simulink model "BLAC_MotorCtrl_Math"  (R2025b)
settings: Solver=FixedStepDiscrete  StartTime=0.0  StopTime=5  FixedStep=MC_Sim_BaseStep  RelTol=1e-3  EnableMultiTasking=on
values from neighbouring files (symbols this model uses):
  MC_Hardware_Chip_ADCResultBit = 0.0    [MotorControlDataDictionary_Math.sldd]
  MC_Hardware_Chip_ADCVoltageMax = 1.0    [MotorControlDataDictionary_Math.sldd]
  MC_Hardware_Chip_ADCVoltageRefence = 0.0    [MotorControlDataDictionary_Math.sldd]
  MC_Hardware_Chip_CSAGain = 1.0    [MotorControlDataDictionary_Math.sldd]
  MC_Sim_BaseStep = 2.5E-8    [MotorControlDataDictionary_Math.sldd]
  MC_Sim_HFTStep = 6.6675E-5    [MotorControlDataDictionary_Math.sldd]
undefined symbols (not defined in the file or in its folder): MC_MOS_DeadTime, MC_Motor_Phi, MC_Motor_Rotor_Pn, MC_Motor_Stator_Ld, MC_Motor_Stator_Lq, MC_Motor_Stator_Rs, MC_Param_CurrentPI_Ki, MC_Param_CurrentPI_Kp, MC_Param_CurrentPI_UdInteMax, MC_Param_CurrentPI_UdInteMin, MC_Param_CurrentPI_UdMax, MC_Param_CurrentPI_UdMin, MC_Param_CurrentPI_UqInteMax, MC_Param_CurrentPI_UqInteMin, MC_Param_CurrentPI_UqMax, MC_Param_CurrentPI_UqMin, MC_Param_Flux_Gamma, MC_Param_Flux_Lalpha, MC_Param_Flux_Lbeta, MC_Param_Flux_Ralpha, MC_Param_Flux_Rbeta, MC_Param_Luen_BEMFalpha, MC_Param_Luen_BEMFbeta, MC_Param_Luen_BEMFErr, MC_Param_Luen_Currentalpha, MC_Param_Luen_Currentbeta, MC_Param_Luen_CurrentErr, MC_Param_Luen_PLL_Ki, MC_Param_Luen_PLL_Kp, MC_Param_Luen_Voltagealpha, MC_Param_Luen_Voltagebeta, MC_Param_PhasetoReal, MC_Param_SMO_CoffA, MC_Param_SMO_CoffB, MC_Param_SpeedtoTheta, MC_Param_SVPWM_DutyMax, MC_Param_SVPWM_DutyMin, MC_Param_SVPWM_SampleOffset1, MC_Param_SVPWM_SampleOffset2, MC_Param_SVPWM_SampleValid
libraries: simulink x31, nesl_utility x22, ee_lib x21, fl_lib x16, spsSeriesRLCBranchLib x2, spsVoltageMeasurementLib x2
(part 1 of 5)
settings Model: DataDictionary=MotorControlDataDictionary_Math.sldd  SimulationMode=accelerator  Creator=YXuan  LastModifiedBy=YXuan
settings SolverCC: PositivePriorityOrder=on  AutoInsertRateTranBlk=on
settings OptimizationCC: DefaultParameterBehavior=Inlined  EnhancedBackFolding=on  PassReuseOutputArgsAs=Individual arguments  ZeroExternalMemoryAtStartup=off  ZeroInternalMemoryAtStartup=off  OptimizeBlockOrder=speed  DifferentSizesBufferReuse=on  OptimizationCustomize=off  EfficientTunableParamExpr=on
settings DebuggingCC: ParameterTunabilityLossMsg=error
settings SFSimCC: MATLABDynamicMemAlloc=off
settings RTWCC: SystemTargetFile=ert.tlc  TemplateMakefile=ert_default_tmf  GPUComputeCapability=3.5  Description=Embedded Coder
settings CodeAppCC: ForceParamTrailComments=on  IgnoreCustomStorageClasses=off  OperatorAnnotations=on  SimulinkDataObjDesc=on  SFDataObjDesc=on  InsertBlockDesc=on
settings ERTTargetCC: ERTCustomFileTemplate=example_file_process.tlc  DynamicArrayContainerType=coder::array  TargetLangStandard=C99 (ISO)  GenerateSampleERTMain=on

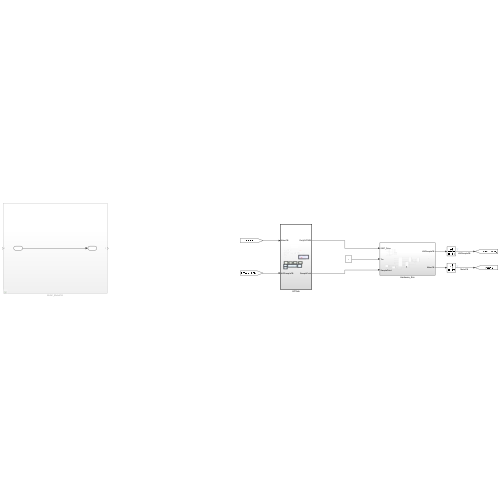
[thumbnail: Simulink's stored preview of the top-level diagram]
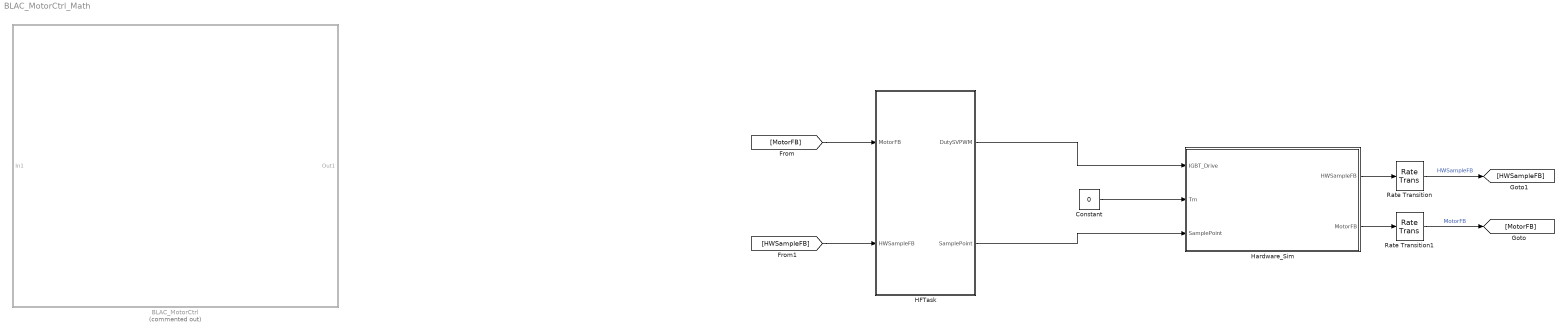
== system BLAC_MotorCtrl_Math ==
  BLAC_MotorCtrl : Subsystem  Commented=on
  Constant : Constant  Value=0
  HFTask : Subsystem  TreatAsAtomicUnit=on  SystemSampleTime=MC_Sim_HFTStep
  Hardware_Sim : Subsystem
  Rate Transition : RateTransition  OutPortSampleTime=MC_Sim_HFTStep
  Rate Transition1 : RateTransition  OutPortSampleTime=MC_Sim_HFTStep
  wires:
  HFTask/1(DutySVPWM) -> Hardware_Sim/1(IGBT_Drive)
  HFTask/2(SamplePoint) -> Hardware_Sim/3(SamplePoint)
  [MotorFB] -> HFTask/1(MotorFB)
  [HWSampleFB] -> HFTask/2(HWSampleFB)
  Constant/1 -> Hardware_Sim/2(Tm)
  Hardware_Sim/2(MotorFB) -> Rate Transition1/1
  Hardware_Sim/1(HWSampleFB) -> Rate Transition/1
  Rate Transition/1 -> [HWSampleFB]  "HWSampleFB"
  Rate Transition1/1 -> [MotorFB]  "MotorFB"

== system BLAC_MotorCtrl_Math/BLAC_MotorCtrl ==
  In1 : Inport
  Out1 : Outport
  wires:
  In1/1 -> Out1/1

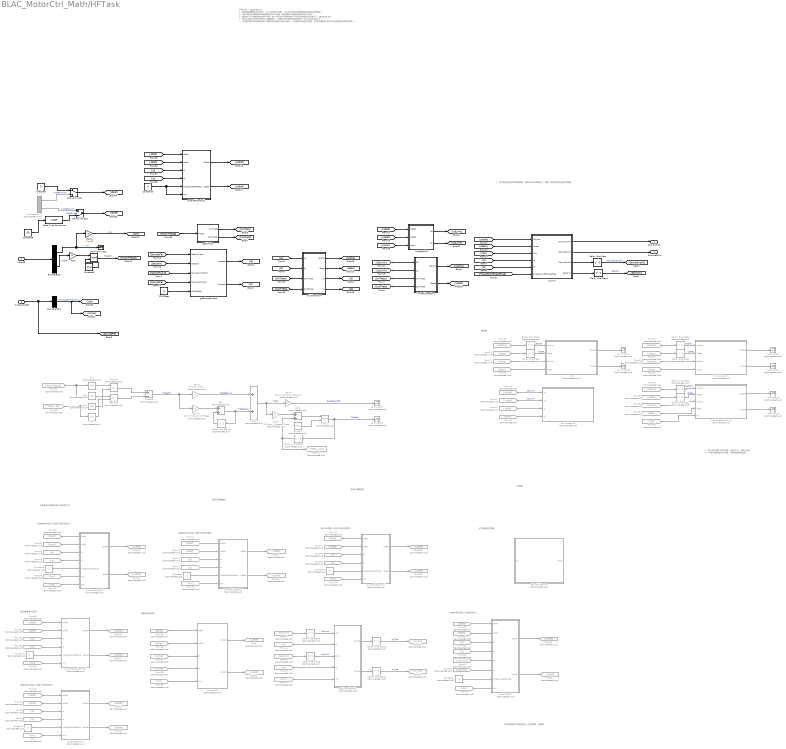
== system BLAC_MotorCtrl_Math/HFTask ==
  note: 待更新电压控制的积分抗饱和方式
  note: 传统电流PI控制（前馈+电流抗饱和）
  note: 1、PLL存在问题(带宽问题，10hz可以，50hz溢出)
      | 2、方程反馈参数存在问题，导致观测角度超前
  note: 观测器
  note: 无差拍电流控制
  note: 开发日志：
      | 2025.03.24:
      | 1、磁链观测器增益应该适中（过小会导致不收敛，过大则会导致观测角度相位超前实际角度）
      | 2、无差拍电流控制是否采用预测电流进行控制？是否要进行旋转反电势的电压补偿？
      | 3、静态电压补偿模型增益如何设置？输入电压是采用理想电压还是采样的电机实际电压？
      | 2025.03.25:
      | 1、测试发现电压和电流呈现2个周期延时，无差拍应考虑做电流预测两个节拍
      | 2025.03.27：
      | 1、无差拍控制应采用延时两个周期的电流和电压进行延时一个周期的电流进行预测，然后用预测电流作为电流控制的反馈电流输入。
      | 2025.12.13:
      | 1、增加真实相电压计算（待添加）
      | 2、考虑MPTA、弱磁、以及MPTV模块的防止位置
      | 2026.01.01：
      | 1、增加卡尔曼滤波模块（未构建）
      | 2、增加PIR控制器（未整定参数）
      | 2026.01.28：
      | 1、发现ADRC的电流观测值初期收敛速度较慢，并且存在稳定的误差。
  note: 复矢量电流PI控制
  note: 传统电流PI控制（前馈+电压抗饱和）
  note: ADRC电流控制（性能待优化）
  note: 传统电流PID控制（前馈+电流抗饱和）
  note: 待进行参数整定
  note: 电流PIR控制（前馈+电流抗饱和）
  note: 待进行参数整定
  note: 卡尔曼滤波观测器
  note: 待构建
  note: 1、优化的单电阻采样移相策略、增加单边采样策略
      | 2、增加三电阻和两电阻采样策略
  note: 电流观测值与实际值存在一定的误差，待解决
  MotorFB : Inport
  HWSampleFB : Inport  Port=2
  Add : Sum  Commented=on
  Add1 : Sum  Commented=on
  Add2 : Sum  Commented=on
  Bus Selector : BusSelector  OutputSignals=w,theta
  Bus Selector1 : BusSelector  OutputSignals=Vbus_Sample_DC
  Bus Selector3 : BusSelector  Commented=on  OutputSignals=IdRefLimit,IqRefLimit
  CSAOffset : Constant  Value=0  OutDataTypeStr=single
  Constant : Constant  Commented=on  Value=2*pi  OutDataTypeStr=single
  Constant{1..5,7} (6 alike) : Constant  Commented=on  Value=0  OutDataTypeStr=boolean
  Constant6 : Constant  Value=2*pi  OutDataTypeStr=single
  Constant8 : Constant  Value=50
  Constant9 : Constant  Value=0  OutDataTypeStr=boolean
  Data Type Conversion : DataTypeConversion  OutDataTypeStr=single  RndMeth=Simplest  SaturateOnIntegerOverflow=off
  Delay One Step : Delay
  Delay One Step1 : Delay
  Delay One Step{8..11} (4 alike) : Delay  Commented=on  DelayLength=1
  Delay One Step12 : Delay  Commented=on  DelayLength=0
  Delay One Step13 : Delay  Commented=on  DelayLength=0
  Delay One Step{2..7} (6 alike) : Delay  Commented=on
  From{,39,46,59,70,75} (6 alike) : From  Commented=on  GotoTag=Wm
  From{10,35,42,50,60,66,71,76} (8 alike) : From  Commented=on  GotoTag=IdRef
  From{11,36,43,51,61,67,72,77} (8 alike) : From  Commented=on  GotoTag=IqRef
  From{2,44,52,62,68,73,78} (7 alike) : From  Commented=on  GotoTag=Id
  From25 : From  Commented=on  GotoTag=Ualpha
  From26 : From  Commented=on  GotoTag=Ubeta
  From27 : From  Commented=on  GotoTag=Ialpha
  From28 : From  Commented=on  GotoTag=Ibeta
  From{3,45,53,63,69,74,79} (7 alike) : From  Commented=on  GotoTag=Iq
  From31 : From  Commented=on  GotoTag=Ualpha
  From32 : From  Commented=on  GotoTag=Ubeta
  From33 : From  Commented=on  GotoTag=Ialpha
  From34 : From  Commented=on  GotoTag=Ibeta
  From37 : From  Commented=on  GotoTag=Id_Pre
  From38 : From  Commented=on  GotoTag=Iq_Pre
  From40 : From  Commented=on  GotoTag=UdRef
  From41 : From  Commented=on  GotoTag=UqRef
  From47 : From  Commented=on  GotoTag=UdLimit
  From48 : From  Commented=on  GotoTag=UqLimit
  From49 : From  Commented=on  GotoTag=We
  From54 : From  Commented=on  GotoTag=Ualpha
  From55 : From  Commented=on  GotoTag=Ubeta
  From56 : From  Commented=on  GotoTag=Ialpha
  From57 : From  Commented=on  GotoTag=Ibeta
  From58 : From  Commented=on  GotoTag=We
  From64 : From  Commented=on  GotoTag=Vdq
  From65 : From  Commented=on  GotoTag=We
  From80 : From  Commented=on  GotoTag=UdLimit
  From81 : From  Commented=on  GotoTag=UqLimit
  From82 : From  Commented=on  GotoTag=Theta_Last
  From83 : From  Commented=on  GotoTag=MotorThetaE
  Gain : Gain  Gain=4  OutDataTypeStr=single
  Gain2 : Gain  Gain=4*pi/30
  Gain3 : Gain  Commented=on  Gain=2*sqrt(2)/2*100
  Gain4 : Gain  Commented=on  Gain=100^2*MC_Sim_HFTStep
  Gain5 : Gain  Commented=on  Gain=MC_Param_SpeedtoTheta  OutDataTypeStr=single  RndMeth=Simplest
  Gain6 : Gain  Commented=on  Gain=30/(pi*MC_Motor_Rotor_Pn)  OutDataTypeStr=single  RndMeth=Simplest
  Goto{,14,30,32,35,37,39} (7 alike) : Goto  Commented=on  GotoTag=UdRef
  Goto{10,26..27,31,34,36,38} (7 alike) : Goto  Commented=on  GotoTag=UqRef
  Goto28 : Goto  Commented=on  GotoTag=Id_Pre
  Goto29 : Goto  Commented=on  GotoTag=Iq_Pre
  Goto40 : Goto  Commented=on  GotoTag=Theta_Last
  Idref_Test : Constant  Value=0  OutDataTypeStr=single
  LuenbergerObservor : Subsystem  Commented=on
  Manual Switch : ManualSwitch
  Manual Switch1 : ManualSwitch  CurrentSetting=0
  Mod : Math  Operator=mod
  Mod1 : Math  Commented=on  Operator=mod
  Product : Product  Commented=on
  Product1 : Product  Commented=on
  Sin : Trigonometry  Commented=on  OutputSignalType=real
  Sin1 : Trigonometry  Commented=on  Operator=cos  OutputSignalType=real
  Sin2 : Trigonometry  Commented=on  OutputSignalType=real
  Sin3 : Trigonometry  Commented=on  Operator=cos  OutputSignalType=real
  Subtract : Sum  Commented=on  Inputs=+-
  Terminator : Terminator
  Terminator{1..8} (8 alike) : Terminator  Commented=on
  axisTransform : Subsystem
  currentADRC : Subsystem  Commented=on
  currentComplexPICtrl : Subsystem  Commented=on
  currentDBC : Subsystem  Commented=on
  currentPIControl : Subsystem  Commented=on
  currentPIControl1 : Subsystem  Commented=on
  currentPIControl2 : Subsystem
  currentPIDControl : Subsystem  Commented=on
  currentPIRControl : Subsystem  Commented=on
  fluxobservor : Subsystem  Commented=on
  getCurrentPredict : Subsystem  Commented=on
  getPhaseCurrent : Subsystem
  getSinCos : Subsystem
  invParkTransform : Subsystem
  karmalObservor : Subsystem  Commented=on
  scvmobservor : Subsystem  Commented=on
  smo : Subsystem  Commented=on
  svpwm : Subsystem  TreatAsAtomicUnit=on
  voltageLimit : Subsystem
  DutySVPWM : Outport
  SamplePoint : Outport  Port=2
  wires:
  Delay One Step2/1 -> smo/1(Valpha)  "Ualpha"
  From25/1 -> Delay One Step2/1
  Delay One Step3/1 -> smo/2(Vbeta)  "Ubeta"
  From26/1 -> Delay One Step3/1
  From27/1 -> smo/3(Ialpha)
  From28/1 -> smo/4(Ibeta)
  smo/1(Speed) -> Terminator2/1
  smo/2(Theta) -> Terminator3/1
  [PhaseShortEnableFlag] -> svpwm/6(PhaseShortEnableFlag)
  [Umax] -> voltageLimit/3(Umax)
  svpwm/4(SectorN) -> Delay One Step1/1
  axisTransform/2(Ibeta) -> [Ibeta]
  svpwm/3(SampleValid) -> Delay One Step/1
  svpwm/1(DutySVPWM) -> DutySVPWM/1
  [SampleFB] -> getPhaseCurrent/4(SampleCurrent)
  [SectorN] -> getPhaseCurrent/2(SectorN)
  [UdRef] -> voltageLimit/1(UdRef)
  [UdLimit] -> invParkTransform/1(Ud)
  currentPIControl/1(UdRef) -> Goto14/1
  [Ubeta] -> svpwm/2(Vbeta)
  axisTransform/1(Ialpha) -> [Ialpha]
  [UqRef] -> voltageLimit/2(UqRef)
  [Ualpha] -> svpwm/1(Valpha)
  [Ia] -> axisTransform/1(Ia)
  svpwm/2(SamplePoint) -> SamplePoint/1
  currentPIControl/2(UqRef) -> Goto10/1
  [Vdc] -> svpwm/3(Vdc)
  voltageLimit/1(Ud) -> [UdLimit]
  [MotorThetaE] -> getSinCos/1(Theta)
  From2/1 -> currentPIControl/3(Id)
  getSinCos/1(SinTheta) -> [SinTheta]
  [SampleValid] -> getPhaseCurrent/3(SampleValid[2])
  axisTransform/3(Id) -> [Id]
  getPhaseCurrent/2(Ibselect) -> [Ib]
  From/1 -> currentPIControl/6(Wm)
  axisTransform/4(Iq) -> [Iq]
  From3/1 -> currentPIControl/4(Iq)
  Constant2/1 -> currentPIControl/5(IntregralResetFlag)
  [Ib] -> axisTransform/2(Ib)
  [UqLimit] -> invParkTransform/2(Uq)
  [SinTheta] -> invParkTransform/3(SinTheta)
  Delay One Step1/1 -> [SectorN]  "SectorN"
  [CosTheta] -> invParkTransform/4(CosTheta)
  invParkTransform/1(Ualpha) -> [Ualpha]
  Delay One Step/1 -> [SampleValid]  "SampleValid[2]"
  getSinCos/2(CosTheta) -> [CosTheta]
  voltageLimit/2(Uq) -> [UqLimit]
  [SinTheta] -> axisTransform/3(SinTheta)
  getPhaseCurrent/1(Iaselect) -> [Ia]
  CSAOffset/1 -> getPhaseCurrent/5(CSAOffset)
  [CosTheta] -> axisTransform/4(CosTheta)
  invParkTransform/2(Ubeta) -> [Ubeta]
  [Ib] -> svpwm/5(Ib)
  [Ia] -> svpwm/4(Ia)
  Bus Selector/2 -> Gain/1  "<theta>"
  Bus Selector/1 -> Terminator/1, Gain2/1  "<w>"
  Mod/1 -> [MotorThetaE]  "ThetaE"
  Gain/1 -> Mod/1
  HWSampleFB/1 -> [SampleFB], Bus Selector1/1
  Constant6/1 -> Mod/2
  MotorFB/1 -> Bus Selector/1
  From10/1 -> currentPIControl/1(IdRef)
  From11/1 -> currentPIControl/2(IqRef)
  From34/1 -> fluxobservor/4(Ibeta)
  From33/1 -> fluxobservor/3(Ialpha)
  From32/1 -> Delay One Step5/1
  From31/1 -> Delay One Step4/1
  Delay One Step4/1 -> fluxobservor/1(Valpha)  "Ualpha"
  Delay One Step5/1 -> fluxobservor/2(Vbeta)  "Ubeta"
  fluxobservor/1(Speed) -> Terminator1/1
  fluxobservor/2(Theta) -> Terminator4/1
  currentDBC/2(UqRef) -> Goto26/1
  From36/1 -> currentDBC/2(IqRef)
  From35/1 -> currentDBC/1(IdRef)
  From37/1 -> currentDBC/3(Id)
  From38/1 -> currentDBC/4(Iq)
  From39/1 -> currentDBC/5(Wm)
  From41/1 -> scvmobservor/2(Vq)  "UqLimit"
  From40/1 -> scvmobservor/1(Vd)  "UdLimit"
  From42/1 -> scvmobservor/3(Id)
  From43/1 -> scvmobservor/4(Iq)
  Gain2/1 -> [We]  "We"
  From44/1 -> getCurrentPredict/2(Id)
  From45/1 -> getCurrentPredict/4(Iq)
  From46/1 -> getCurrentPredict/5(Wm)
  From47/1 -> Delay One Step8/1
  From48/1 -> Delay One Step9/1
  getCurrentPredict/1(Id_Pre) -> Delay One Step12/1
  getCurrentPredict/2(Iq_Pre) -> Delay One Step13/1
  currentDBC/1(UdRef) -> Goto/1
  Delay One Step8/1 -> getCurrentPredict/1(Ud1)  "UdLimit"
  Delay One Step9/1 -> getCurrentPredict/3(Uq1)  "UqLimit"
  Delay One Step12/1 -> Goto28/1  "Id_Pre"
  Delay One Step13/1 -> Goto29/1  "Iq_Pre"
  From51/1 -> currentComplexPICtrl/2(IqRef)
  From50/1 -> currentComplexPICtrl/1(IdRef)
  Constant1/1 -> currentComplexPICtrl/5(IntregralResetFlag)
  From53/1 -> currentComplexPICtrl/4(Iq)
  From49/1 -> currentComplexPICtrl/6(Wm)
  From52/1 -> currentComplexPICtrl/3(Id)
  currentComplexPICtrl/2(UqRef) -> Goto27/1
  currentComplexPICtrl/1(UdRef) -> Goto30/1
  LuenbergerObservor/1(Speed) -> Terminator5/1
  LuenbergerObservor/2(Theta) -> Terminator6/1
  From57/1 -> LuenbergerObservor/4(Ibeta)
  From56/1 -> LuenbergerObservor/3(Ialpha)
  From55/1 -> Delay One Step7/1
  From54/1 -> Delay One Step6/1
  Delay One Step7/1 -> LuenbergerObservor/2(Vbeta)  "Ubeta"
  Delay One Step6/1 -> LuenbergerObservor/1(Valpha)  "Ualpha"
  From58/1 -> LuenbergerObservor/5(We)
  From61/1 -> currentPIControl1/2(IqRef)
  From60/1 -> currentPIControl1/1(IdRef)
  Constant3/1 -> currentPIControl1/5(IntregralResetFlag)
  From63/1 -> currentPIControl1/4(Iq)
  From59/1 -> currentPIControl1/6(Wm)
  From62/1 -> currentPIControl1/3(Id)
  currentPIControl1/2(UqRef) -> Goto31/1
  currentPIControl1/1(UdRef) -> Goto32/1
  From64/1 -> currentPIControl1/7(Vdq)
  currentADRC/1(UdRef) -> Goto35/1
  currentADRC/2(UqRef) -> Goto34/1
  From68/1 -> currentADRC/3(Id)
  From65/1 -> currentADRC/8(Wm)
  From69/1 -> currentADRC/4(Iq)
  Constant4/1 -> currentADRC/7(IntregralResetFlag)
  From66/1 -> currentADRC/1(IdRef)
  From67/1 -> currentADRC/2(IqRef)
  Constant5/1 -> currentPIDControl/5(IntregralResetFlag)
  From71/1 -> currentPIDControl/1(IdRef)
  currentPIDControl/1(UdRef) -> Goto37/1
  From73/1 -> currentPIDControl/3(Id)
  From72/1 -> currentPIDControl/2(IqRef)
  currentPIDControl/2(UqRef) -> Goto36/1
  From70/1 -> currentPIDControl/6(Wm)
  From74/1 -> currentPIDControl/4(Iq)
  Bus Selector3/1 -> Manual Switch/2  "<IdRefLimit>"
  Bus Selector3/2 -> Manual Switch1/1  "<IqRefLimit>"
  Manual Switch/1 -> [IdRef]
  Idref_Test/1 -> Manual Switch/1
  Manual Switch1/1 -> [IqRef]
  Data Type Conversion/1 -> Manual Switch1/2  "IqRef_Test"
  From79/1 -> currentPIRControl/4(Iq)
  From75/1 -> currentPIRControl/6(Wm)
  currentPIRControl/2(UqRef) -> Goto38/1
  From77/1 -> currentPIRControl/2(IqRef)
  From78/1 -> currentPIRControl/3(Id)
  currentPIRControl/1(UdRef) -> Goto39/1
  From76/1 -> currentPIRControl/1(IdRef)
  Constant7/1 -> currentPIRControl/5(IntregralResetFlag)
  From80/1 -> currentADRC/5(Ud)
  From81/1 -> currentADRC/6(Uq)
  Gain5/1 -> Add2/1
  Delay One Step10/1 -> Add/2
  Constant/1 -> Mod1/2
  Mod1/1 -> Terminator8/1, Delay One Step11/1  "ThetaPI"
  Delay One Step11/1 -> Goto40/1, Add2/2
  Gain3/1 -> Add1/1  "ThetaErr_Kp"
  Add1/1 -> Gain6/1, Gain5/1  "WePI"
  Add2/1 -> Mod1/1
  Gain6/1 -> Terminator7/1  "SpeedPI_RPM"
  Subtract/1 -> Gain3/1, Gain4/1  "ThetaErr"
  Add/1 -> Add1/2, Delay One Step10/1  "ThetaErr_Ki"
  Gain4/1 -> Add/1
  From83/1 -> Sin1/1, Sin/1
  From82/1 -> Sin2/1, Sin3/1
  Sin/1 -> Product/1
  Sin3/1 -> Product/2
  Product/1 -> Subtract/1
  Sin1/1 -> Product1/1
  Sin2/1 -> Product1/2
  Product1/1 -> Subtract/2
  Constant8/1 -> Data Type Conversion/1
  [SampleFB] -> getPhaseCurrent/1(RealCurrent)
  Bus Selector1/1 -> [Umax], [Vdc]  "<Vbus_Sample_DC>"
  [IqRef] -> currentPIControl2/2(IqRef)
  [IdRef] -> currentPIControl2/1(IdRef)
  [Iq] -> currentPIControl2/4(Iq)
  [Id] -> currentPIControl2/3(Id)
  currentPIControl2/2(UqRef) -> [UqRef]
  currentPIControl2/1(UdRef) -> [UdRef]
  Constant9/1 -> currentPIControl2/6(Wm), currentPIControl2/5(IntregralResetFlag)

== system BLAC_MotorCtrl_Math/Hardware_Sim ==
  IGBT_Drive : Inport
  Tm : Inport  Port=2
  SamplePoint : Inport  Port=3
  ActoDC_Sim : Subsystem
      settings: PortSchema="{\"entries\":[{\"content\":{\"sides\":[{\"content\":{},\"type\":\"ConnectorPlacement.EquallySpacedRectSide\",\"uuid\":\"dfb3aeea-336c-446c-ad65-e2bc7f8ca636\"},{\"content\":{\"connectorIds\":[\"RConn1\",\"RConn2\",\"RConn3\",\"RConn4\"],\"side\":\"RIGHT\"},\"type\":\"ConnectorPlacement.EquallySpacedRectSide\",\"uuid\":\"0d159b54-293a-4c78-aa60-b1815773a2e6\"},{\"content\":{\"side\":\"TOP\"},\"type\":\"ConnectorPlacement.EquallySpacedRectSide\",\"uuid\":\"3a8a1089-02f9-49de-abe1-3c0c9b1c30b4\"},{\"content\":{\"connectorIds\":[\"RConn5\"],\"side\":\"BOTTOM\"},\"type\":\"ConnectorPlacement.EquallySpacedRectSide\",\"uuid\":\"d5f8019e-9277-4fe4-88e1-78a5ead24f5f\"}]},\"type\":\"ConnectorPlacement.EquallySpacedConnector\",\"uuid\":\"60ec8383-903f-4624-bd14-64a171abc59f\"}],\"packageUris\":[\"http://schema.mathworks.com/mf0/Connector/R2020b\"],\"version\":\"1.0\"}"
  CurrentSample_Sim : Subsystem
      settings: PortSchema="{\"entries\":[{\"content\":{\"sides\":[{\"content\":{\"connectorIds\":[\"LConn1\",\"LConn2\",\"LConn3\"]},\"type\":\"ConnectorPlacement.EquallySpacedRectSide\",\"uuid\":\"6ff7a8d3-c405-46c2-bb14-4046cb7aeae7\"},{\"content\":{\"connectorIds\":[\"Out1\"],\"side\":\"RIGHT\"},\"type\":\"ConnectorPlacement.EquallySpacedRectSide\",\"uuid\":\"30142a9b-9a7e-41fc-b1d2-e3039139c6ca\"},{\"content\":{\"connectorIds\":[\"In1\"],\"side\":\"TOP\"},\"type\":\"ConnectorPlacement.EquallySpacedRectSide\",\"uuid\":\"3160108e-a18c-4d1a-9078-164fb8c05fb9\"},{\"content\":{\"connectorIds\":[\"RConn1\"],\"side\":\"BOTTOM\"},\"type\":\"ConnectorPlacement.EquallySpacedRectSide\",\"uuid\":\"3a8083c0-8ece-4c47-8031-bf566ef0bce5\"}]},\"type\":\"ConnectorPlacement.EquallySpacedConnector\",\"uuid\":\"b4e632a6-7f3d-4ba3-a4f0-ad8004e8ab56\"}],\"packageUris\":[\"http://schema.mathworks.com/mf0/Connector/R2020b\"],\"version\":\"1.0\"}"
  DrivePWM_Sim : Subsystem
  IGBT_Inverter_Sim : Subsystem
  Motor_Machine_Sim : Subsystem
  PMSM : ee_lib/Electromechanical/Permanent Magnet/PMSM  port_option=ee.enum.threePhasePort.expanded  winding_type=ee.enum.electromech.statorconfiguration.wye  machine_param=ee.enum.pmsm.parameterization.constant  nPolePairs=6  pmflux_param=ee.enum.pmflux.fluxlinkage  pm_flux_linkage=0.03 Wb  torque_constant=0.18 N*m/A  back_emf_constant=0.18 V*s/rad  stator_param=ee.enum.statorparam.LdLqL0  Ld=0.00019 H  Lq=0.00025 H  idVec=[-200, 0, 200] A  iqVec=[-200, 0, 200] A  LdMatrix=0.0002 * ones(3, 3) H  LqMatrix=0.0002 * ones(3, 3) H  PmMatrix=0.1 * ones(3, 3) Wb  ktMatrix=0.18 * ones(3, 3) N*m/A  keMatrix=0.18 * ones(3, 3) V*s/rad  L0=0.00016 H  Ls=0.0002 H  Lm=-0.00002 H  Ms=0.00002 H  Rs=0.013 Ohm  zero_sequence=ee.enum.park.zerosequence.include  axes_param=ee.enum.rotorangle.daxis  loss_param=ee.enum.ironloss.none  losses_oc=[0, 0, 0] W  losses_sc=[0, 0, 0] W  f_losses=60 Hz  Isc_losses=95 A  J=0.01 kg*m^2  lam=0 N*m*s/rad  i_d_specify=off  i_d_priority=None  i_d=0 A  i_d_nominal_specify=off  i_d_nominal_value=1  i_d_nominal_unit=A  i_q_specify=off  i_q_priority=None  i_q=0 A  i_q_nominal_specify=off  i_q_nominal_value=1  i_q_nominal_unit=A  torque_specify=off  torque_priority=None  torque=0 N*m  torque_nominal_specify=off  torque_nominal_value=1  torque_nominal_unit=N*m  angular_velocity_specify=off  angular_velocity_priority=High  angular_velocity=0 rpm  angular_velocity_nominal_specify=off  angular_velocity_nominal_value=1  angular_velocity_nominal_unit=rpm  angular_position_specify=off  angular_position_priority=High  angular_position=0 deg  angular_position_nominal_specify=off  angular_position_nominal_value=1  angular_position_nominal_unit=deg  alpha=3.93e-3 1/K  alpha_flux=-0.001 1/K  Tmeas=298.15 K  stator_thermal_mass=100 J/K  rotor_thermal_mass=200 J/K  Rm_percent_rotor=90  Rd_percent_rotor=30  temperatureA_specify=off  temperatureA_priority=High  temperatureA=25 degC  temperatureA_nominal_specify=off  temperatureA_nominal_value=1  temperatureA_nominal_unit=degC  temperatureB_specify=off  temperatureB_priority=High  temperatureB=25 degC  temperatureB_nominal_specify=off  temperatureB_nominal_value=1  temperatureB_nominal_unit=degC  temperatureC_specify=off  temperatureC_priority=High  temperatureC=25 degC  temperatureC_nominal_specify=off  temperatureC_nominal_value=1  temperatureC_nominal_unit=degC  temperatureR_specify=off  temperatureR_priority=High  temperatureR=25 degC  temperatureR_nominal_specify=off  temperatureR_nominal_value=1  temperatureR_nominal_unit=degC
      settings: InternalSimscapePortConfiguration="{\"Bottom\":[],\"Left\":[{\"id\":\"a\",\"label\":\"a\",\"type\":\"foundation.electrical.electrical\"},{\"id\":\"b\",\"label\":\"b\",\"type\":\"foundation.electrical.electrical\"},{\"id\":\"c\",\"label\":\"c\",\"type\":\"foundation.electrical.electrical\"},{\"id\":\"n\",\"label\":\"n\",\"type\":\"foundation.electrical.electrical\"}],\"Right\":[{\"id\":\"R\",\"label\":\"R\",\"type\":\"foundation.mechanical.rotational.rotational\"},{\"id\":\"C\",\"label\":\"C\",\"type\":\"foundation.mechanical.rotational.rotational\"}],\"Top\":[]}"
  Repeating Sequence : simulink/Sources/Repeating Sequence  rep_seq_t=[0 MC_Sim_HFTStep/2 MC_Sim_HFTStep]  rep_seq_y=[0 1 0]
  SampleTrigger_Sim : Subsystem
  Solver Configuration : nesl_utility/Solver Configuration  PhysicalDomain=network_engine_domain  SubClassName=solver  LeftPortType=input  RightPortType=generic  Tones=[]  Harmonics=[]  SimulateNoise=off  Profile=off  UseLocalSampling=off  EnableSwitchedLinearOptims=on  FrequencyDomain=off  UseCCode=off  RelTol=0.001  AbsTol=0.001  MinStep=1e-09  ToWorkspace=off  RevertToSquareIcSolve=off  NumHomotopyIterations=100  PhasorMode=off  PhasorModeNumHarmonics=1  ConsistencySolver=NEWTON_XTOL_AFTER_FTOL  IndexReductionMethod=DerivativeReplacement  DoDC=off  ResidualTolerance=1e-09  ConsistencyTolSource=GLOBAL  ConsistencyAbsTol=0.001  ConsistencyRelTol=0.001  ConsistencyTolFactor=0.001  UseLocalSolver=off  LocalSolverChoice=NE_BACKWARD_EULER_ADVANCER  ResolveIndetEquations=on  FunctionEvalNumThread=1  LocalSolverSampleTime=0.001  DoFixedCost=off  MaxNonlinIter=3  MaxModeIter=2  ComputeImpulses=off  ImpulseIterations=2  LinearAlgebra=auto  LinearAlgebraNumThread=0  EquationFormulation=NE_TIME_EF  DelaysMemoryBudget=1024  AutomaticFiltering=on  FilteringTimeConstant=0.001  PartitionStorageMethod=AS_NEEDED  PartitionMemoryBudget=1024  PartitionMethod=ROBUST  MultibodyUseLocalSolver=off  MultibodyLocalSolverChoice=ODE1  MultibodyLocalSolverSampleTime=0.001
  Subsystem : Subsystem
      settings: PortSchema="{\"entries\":[{\"content\":{\"sides\":[{\"content\":{\"connectorIds\":[\"LConn1\",\"LConn2\",\"LConn3\"]},\"type\":\"ConnectorPlacement.EquallySpacedRectSide\",\"uuid\":\"af0e302a-6fe8-4ee5-ad7b-36fa2462e52a\"},{\"content\":{\"connectorIds\":[\"Out1\",\"Out2\",\"Out3\",\"RConn1\",\"RConn2\",\"RConn3\",\"RConn4\"],\"side\":\"RIGHT\"},\"type\":\"ConnectorPlacement.EquallySpacedRectSide\",\"uuid\":\"81cc88e0-41b7-4998-ab4b-7cd10d736f31\"},{\"content\":{\"side\":\"TOP\"},\"type\":\"ConnectorPlacement.EquallySpacedRectSide\",\"uuid\":\"a12e26d5-ba08-4fd7-9848-733d0ad7d51d\"},{\"content\":{\"connectorIds\":[\"RConn5\"],\"side\":\"BOTTOM\"},\"type\":\"ConnectorPlacement.EquallySpacedRectSide\",\"uuid\":\"d3c07252-42de-4432-99bf-cb622f01e596\"}]},\"type\":\"ConnectorPlacement.EquallySpacedConnector\",\"uuid\":\"b6ff19e2-c175-4441-b83d-f6984fbd2671\"}],\"packageUris\":[\"http://schema.mathworks.com/mf0/Connector/R2020b\"],\"version\":\"1.0\"}"
  VbusSample_Sim : Subsystem
      settings: PortSchema="{\"entries\":[{\"content\":{\"sides\":[{\"content\":{\"connectorIds\":[\"LConn1\",\"LConn2\",\"LConn3\",\"LConn4\"]},\"type\":\"ConnectorPlacement.EquallySpacedRectSide\",\"uuid\":\"516f667a-d28d-4d7e-bf09-1844ec397ca8\"},{\"content\":{\"connectorIds\":[\"Out1\",\"Out2\"],\"side\":\"RIGHT\"},\"type\":\"ConnectorPlacement.EquallySpacedRectSide\",\"uuid\":\"8e4c85e3-3d11-4eb4-88a0-2693c28d829e\"},{\"content\":{\"connectorIds\":[\"In1\"],\"side\":\"TOP\"},\"type\":\"ConnectorPlacement.EquallySpacedRectSide\",\"uuid\":\"147b6efa-5ce1-4794-b48d-7dda172e67f0\"}]},\"type\":\"ConnectorPlacement.EquallySpacedConnector\",\"uuid\":\"ecacdeaf-2c45-44a5-a2ad-63e6b49d0bd0\"}],\"packageUris\":[\"http://schema.mathworks.com/mf0/Connector/R2020b\"],\"version\":\"1.0\"}"
  HWSampleFB : Outport
  MotorFB : Outport  Port=2
  wires:
  CurrentSample_Sim/1(Current_Sample) -> [Current_Sample]
  VbusSample_Sim/1(Vbus_Sample_AC) -> [Vbus_Sample_AC]
  VbusSample_Sim/2(Vbus_Sample_DC) -> [Vbus_Sample_DC]
  SamplePoint/1 -> SampleTrigger_Sim/2(SamplePoint)
  Repeating Sequence/1 -> SampleTrigger_Sim/1(ClockCounter), DrivePWM_Sim/1(ClockCounter)
  IGBT_Drive/1 -> DrivePWM_Sim/2(DrivePWM)
  DrivePWM_Sim/1(Drive_A) -> [Drive_A]
  DrivePWM_Sim/2(Drive_B) -> [Drive_B]
  DrivePWM_Sim/3(Drive_C) -> [Drive_C]
  SampleTrigger_Sim/1(Current_Sample_Trigger) -> [Current_Sample_Trigger]
  SampleTrigger_Sim/2(Vbus_Sample_Trigger) -> [Vbus_Sample_Trigger]
  SampleTrigger_Sim/3(Temp_Sample_Trigger) -> [Temp_Sample_Trigger]
  [Vbus_Sample_Trigger] -> VbusSample_Sim/1(Vbus_Sample_Trigger)
  Tm/1 -> [MotorLoad]
  [Current_Sample_Trigger] -> CurrentSample_Sim/1(Current_Sample_Trigger)
  [Drive_A] -> IGBT_Inverter_Sim/1(DriveA)
  [Drive_B] -> IGBT_Inverter_Sim/2(DriveB)
  [Drive_C] -> IGBT_Inverter_Sim/3(DriveC)
  connections:
  PMSM/RConn1 -- Motor_Machine_Sim/LConn1
  PMSM/RConn2 -- Motor_Machine_Sim/LConn2 -- Solver Configuration/RConn1
  Subsystem/RConn1 -- PMSM/LConn1
  Subsystem/RConn2 -- PMSM/LConn2
  Subsystem/RConn3 -- PMSM/LConn3
  PMSM/LConn4 -- Subsystem/RConn4
  IGBT_Inverter_Sim/RConn1 -- Subsystem/LConn1
  IGBT_Inverter_Sim/RConn2 -- Subsystem/LConn2
  IGBT_Inverter_Sim/RConn3 -- Subsystem/LConn3
  VbusSample_Sim/LConn1 -- ActoDC_Sim/RConn1 -- IGBT_Inverter_Sim/LConn1
  VbusSample_Sim/LConn2 -- ActoDC_Sim/RConn2
  VbusSample_Sim/LConn3 -- ActoDC_Sim/RConn3
  VbusSample_Sim/LConn4 -- ActoDC_Sim/RConn4
  IGBT_Inverter_Sim/RConn4 -- CurrentSample_Sim/LConn1
  IGBT_Inverter_Sim/RConn5 -- CurrentSample_Sim/LConn2
  IGBT_Inverter_Sim/RConn6 -- CurrentSample_Sim/LConn3
  Subsystem/RConn5 -- CurrentSample_Sim/RConn1 -- ActoDC_Sim/RConn5

== system BLAC_MotorCtrl_Math/HFTask/LuenbergerObservor ==
  Valpha : Inport
  Vbeta : Inport  Port=2
  Ialpha : Inport  Port=3
  Ibeta : Inport  Port=4
  We : Inport  Port=5
  Delay One Step : Delay  DelayLength=1  InitialCondition=single(0)
  Terminator : Terminator
  getE : Subsystem
  getSpeedandTheta : Subsystem
  Speed : Outport
  Theta : Outport  Port=2
  wires:
  getSpeedandTheta/2(Theta) -> Theta/1
  getSpeedandTheta/1(Speed) -> Speed/1
  getE/2(Ebeta) -> getSpeedandTheta/2(Ebeta)
  getE/1(Ealpha) -> getSpeedandTheta/1(Ealpha)
  Ibeta/1 -> getE/4(Ibeta)
  Ialpha/1 -> getE/3(Ialpha)
  Vbeta/1 -> getE/2(Vbeta)
  Valpha/1 -> getE/1(Valpha)
  getSpeedandTheta/3(We) -> Delay One Step/1
  We/1 -> Terminator/1
  Delay One Step/1 -> getE/5(We)

== system BLAC_MotorCtrl_Math/HFTask/axisTransform ==
  Ia : Inport
  Ib : Inport  Port=2
  SinTheta : Inport  Port=3
  CosTheta : Inport  Port=4
  Add1 : Sum
  Product{,1..3} (4 alike) : Product
  Signal Copy : SignalConversion  OverrideOpt=off
  Subtract : Sum  Inputs=-+
  a_plus_2b : Sum  Inputs=+++  RndMeth=Simplest  OutDataTypeStr=Inherit: Same as first input
  one_by_sqrt3 : Gain  Gain=1/sqrt(3)  RndMeth=Simplest  OutDataTypeStr=Inherit: Same as input
  Ialpha : Outport
  Ibeta : Outport  Port=2
  Id : Outport  Port=3
  Iq : Outport  Port=4
  wires:
  Product3/1 -> Subtract/2
  Product2/1 -> Subtract/1
  Add1/1 -> Id/1  "Id"
  Subtract/1 -> Iq/1  "Iq"
  Product/1 -> Add1/1
  Product1/1 -> Add1/2
  CosTheta/1 -> Product3/2, Product/2
  SinTheta/1 -> Product2/2, Product1/2
  a_plus_2b/1 -> one_by_sqrt3/1
  one_by_sqrt3/1 -> Ibeta/1, Product3/1, Product1/1  "Ibeta"
  Signal Copy/1 -> Ialpha/1, Product2/1, Product/1  "Ialpha"
  Ia/1 -> a_plus_2b/1, Signal Copy/1
  Ib/1 -> a_plus_2b/3, a_plus_2b/2

== system BLAC_MotorCtrl_Math/HFTask/currentADRC ==
  note: ADRC开发日志:
      | 20251229：
      | 感觉观测器参数存在问题，观测值瞬间会和参考值相等，导致PI控制器调节电流增速较慢
      | 2026.01.05
      | 1、LESO中的两个fal函数出现周期性震荡
      | 2、NLSEF中的电压输出值只有1.xV，电机转速无法提升
      | 2026.01.07
      | 1、减小NLSEF的参数，可以实现系统的收敛，且效果与PI控制器类似
  IdRef : Inport
  IqRef : Inport  Port=2
  Id : Inport  Port=3
  Iq : Inport  Port=4
  Ud : Inport  Port=5
  Uq : Inport  Port=6
  IntregralResetFlag : Inport  Port=7
  Wm : Inport  Port=8
  Delay One Step : Delay  InitialCondition=single(0)
  Delay One Step1 : Delay  InitialCondition=single(0)
  LESO : Subsystem  VariantControl=ESO
  NLSEF : Subsystem  VariantControl=NLSEF
  Terminator : Terminator
  UdRef : Outport
  UqRef : Outport  Port=2
  wires:
  NLSEF/1(Ud_ADRC) -> UdRef/1  "UdRef"
  NLSEF/2(Uq_ADRC) -> UqRef/1  "UqRef"
  IdRef/1 -> NLSEF/1(Id_Ref)
  Id/1 -> LESO/1(Id)
  IqRef/1 -> NLSEF/2(Iq_Ref)
  Iq/1 -> LESO/3(Iq)
  IntregralResetFlag/1 -> Terminator/1
  Delay One Step/1 -> LESO/2(Ud)
  Delay One Step1/1 -> LESO/4(Uq)
  LESO/2(Iq_ESO) -> NLSEF/4(Iq_ESO)
  LESO/1(Id_ESO) -> NLSEF/3(Id_ESO)
  LESO/3(Id_Dis) -> NLSEF/5(Id_ESO_Dis)
  LESO/4(Iq_Dis) -> NLSEF/6(Iq_ESO_Dis)
  Ud/1 -> Delay One Step/1
  Uq/1 -> Delay One Step1/1

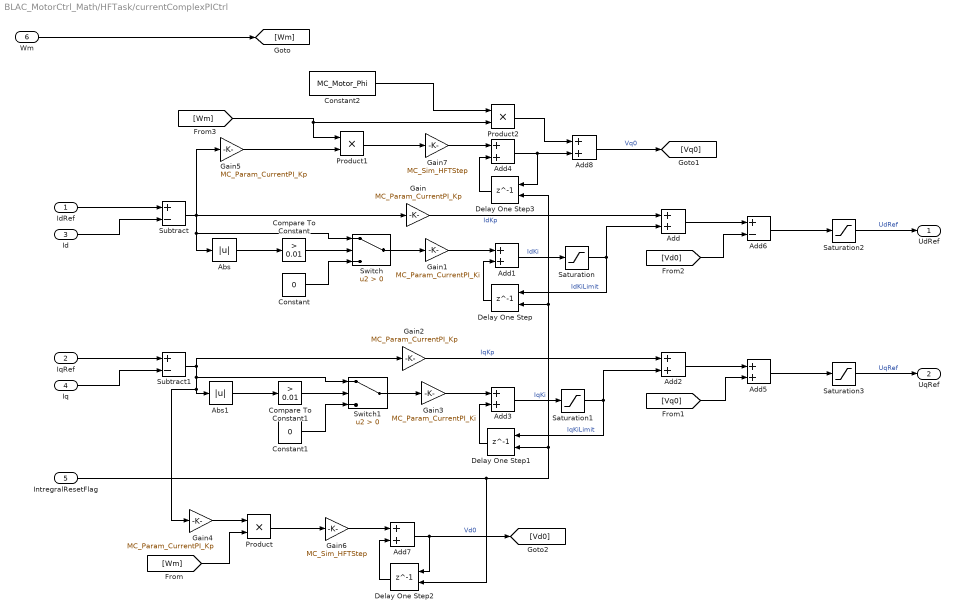
== system BLAC_MotorCtrl_Math/HFTask/currentComplexPICtrl ==
  IdRef : Inport
  IqRef : Inport  Port=2
  Id : Inport  Port=3
  Iq : Inport  Port=4
  IntregralResetFlag : Inport  Port=5
  Wm : Inport  Port=6
  Abs : Abs  SaturateOnIntegerOverflow=off
  Abs1 : Abs  SaturateOnIntegerOverflow=off
  Add{,2,5,8} (4 alike) : Sum
  Add{1,3..4,7} (4 alike) : Sum  OutDataTypeStr=single
  Add6 : Sum  Inputs=+-
  Compare To Constant : simulink/Logic and Bit Operations/Compare To Constant  relop=>  const=0.01  OutDataTypeStr=boolean
  Compare To Constant1 : simulink/Logic and Bit Operations/Compare To Constant  relop=>  const=0.01  OutDataTypeStr=boolean
  Constant : Constant  Value=0  OutDataTypeStr=single
  Constant1 : Constant  Value=0  OutDataTypeStr=single
  Constant2 : Constant  Value=MC_Motor_Phi  OutDataTypeStr=single
  Delay One Step{,1..3} (4 alike) : Delay  DelayLength=1  ExternalReset=Level
      settings: InputPortMap=u0,r5
  Gain : Gain  Gain=MC_Param_CurrentPI_Kp  OutDataTypeStr=single
  Gain1 : Gain  Gain=MC_Param_CurrentPI_Ki  OutDataTypeStr=single
  Gain2 : Gain  Gain=MC_Param_CurrentPI_Kp  OutDataTypeStr=single
  Gain3 : Gain  Gain=MC_Param_CurrentPI_Ki  OutDataTypeStr=single
  Gain4 : Gain  Gain=MC_Param_CurrentPI_Kp
  Gain5 : Gain  Gain=MC_Param_CurrentPI_Kp
  Gain6 : Gain  Gain=MC_Sim_HFTStep  OutDataTypeStr=single
  Gain7 : Gain  Gain=MC_Sim_HFTStep  OutDataTypeStr=single
  Product : Product
  Product1 : Product
  Product2 : Product
  Saturation : Saturate  UpperLimit=MC_Param_CurrentPI_UdInteMax  LowerLimit=MC_Param_CurrentPI_UdInteMin
  Saturation1 : Saturate  UpperLimit=MC_Param_CurrentPI_UqInteMax  LowerLimit=MC_Param_CurrentPI_UqInteMin
  Saturation2 : Saturate  UpperLimit=MC_Param_CurrentPI_UdMax  LowerLimit=MC_Param_CurrentPI_UdMin
  Saturation3 : Saturate  UpperLimit=MC_Param_CurrentPI_UqMax  LowerLimit=MC_Param_CurrentPI_UqMin
  Subtract : Sum  Inputs=+-
  Subtract1 : Sum  Inputs=+-
  Switch : Switch  Criteria=u2 > Threshold  SaturateOnIntegerOverflow=off  InputSameDT=off
  Switch1 : Switch  Criteria=u2 > Threshold  SaturateOnIntegerOverflow=off  InputSameDT=off
  UdRef : Outport
  UqRef : Outport  Port=2
  wires:
  Wm/1 -> [Wm]
  Saturation3/1 -> UqRef/1  "UqRef"
  Saturation2/1 -> UdRef/1  "UdRef"
  [Vd0] -> Add6/2
  Add6/1 -> Saturation2/1
  Add/1 -> Add6/1
  [Vq0] -> Add5/2
  Add2/1 -> Add5/1
  [Wm] -> Product/2
  Id/1 -> Subtract/2
  Gain4/1 -> Product/1
  Switch1/1 -> Gain3/1
  Abs1/1 -> Compare To Constant1/1
  Compare To Constant1/1 -> Switch1/2
  Constant1/1 -> Switch1/3
  Constant/1 -> Switch/3
  Compare To Constant/1 -> Switch/2
  Switch/1 -> Gain1/1
  Add5/1 -> Saturation3/1
  IqRef/1 -> Subtract1/1
  Iq/1 -> Subtract1/2
  Subtract1/1 -> Gain2/1, Gain4/1, Abs1/1, Switch1/1
  Gain2/1 -> Add2/1  "IqKp"
  Gain3/1 -> Add3/1
  Delay One Step1/1 -> Add3/2
  Add3/1 -> Saturation1/1  "IqKi"
  Saturation1/1 -> Add2/2, Delay One Step1/1  "IqKiLimit"
  Saturation/1 -> Delay One Step/1, Add/2  "IdKiLimit"
  Add1/1 -> Saturation/1  "IdKi"
  Delay One Step/1 -> Add1/2
  Gain1/1 -> Add1/1
  Abs/1 -> Compare To Constant/1
  Gain/1 -> Add/1  "IdKp"
  Subtract/1 -> Gain5/1, Abs/1, Switch/1, Gain/1
  IdRef/1 -> Subtract/1
  Gain6/1 -> Add7/1
  Product/1 -> Gain6/1
  Delay One Step2/1 -> Add7/2
  Add7/1 -> [Vd0], Delay One Step2/1  "Vd0"
  Add4/1 -> Delay One Step3/1, Add8/2
  Delay One Step3/1 -> Add4/2
  Gain7/1 -> Add4/1
  IntregralResetFlag/1 -> Delay One Step2/2, Delay One Step1/2, Delay One Step3/2, Delay One Step/2
  Product1/1 -> Gain7/1
  Constant2/1 -> Product2/1
  Gain5/1 -> Product1/2
  Add8/1 -> [Vq0]  "Vq0"
  Product2/1 -> Add8/1
  [Wm] -> Product1/1, Product2/2

== system BLAC_MotorCtrl_Math/HFTask/currentDBC ==
  note: 无差拍电流控制器（延时1拍）
  IdRef : Inport
  IqRef : Inport  Port=2
  Id : Inport  Port=3
  Iq : Inport  Port=4
  Wm : Inport  Port=5
  Add5 : Sum  Inputs=++-
  Add6 : Sum  Inputs=+++
  Add7 : Sum
  Constant1 : Constant  Value=MC_Motor_Phi  OutDataTypeStr=single
  Gain10 : Gain  Gain=MC_Motor_Stator_Lq
  Gain11 : Gain  Gain=MC_Motor_Stator_Lq/MC_Sim_HFTStep
  Gain12 : Gain  Gain=MC_Motor_Stator_Rs-(MC_Motor_Stator_Lq/MC_Sim_HFTStep)
  Gain13 : Gain  Gain=MC_Motor_Stator_Ld
  Gain8 : Gain  Gain=MC_Motor_Stator_Ld/MC_Sim_HFTStep
  Gain9 : Gain  Gain=MC_Motor_Stator_Rs-(MC_Motor_Stator_Ld/MC_Sim_HFTStep)
  Product2 : Product
  Product3 : Product
  Saturation : Saturate  UpperLimit=MC_Param_CurrentPI_UdMax  LowerLimit=MC_Param_CurrentPI_UdMin
  Saturation1 : Saturate  UpperLimit=MC_Param_CurrentPI_UqMax  LowerLimit=MC_Param_CurrentPI_UqMin
  UdRef : Outport
  UqRef : Outport  Port=2
  wires:
  Wm/1 -> [Wm]
  Iq/1 -> [Iq]
  Id/1 -> [Id]
  IqRef/1 -> [IqRef]
  IdRef/1 -> [IdRef]
  [IdRef] -> Gain8/1
  Gain8/1 -> Add5/1  "IdRef_Vd"
  [Id] -> Gain9/1
  Gain9/1 -> Add5/2  "Id_Vd"
  [Iq] -> Gain10/1
  Gain10/1 -> Product2/2
  [Wm] -> Product2/1
  [IqRef] -> Gain11/1
  Gain11/1 -> Add6/1  "IqRef_Vq"
  Gain12/1 -> Add6/2  "Iq_Vq"
  [Iq] -> Gain12/1
  [Wm] -> Product3/1
  Add7/1 -> Product3/2
  Constant1/1 -> Add7/2
  Gain13/1 -> Add7/1
  [Id] -> Gain13/1
  Saturation/1 -> UdRef/1  "UdRef_DBC"
  Saturation1/1 -> UqRef/1  "UqRef_DBC"
  Add5/1 -> Saturation/1
  Product2/1 -> Add5/3  "Iq_Vd"
  Add6/1 -> Saturation1/1
  Product3/1 -> Add6/3  "Id_Vq"

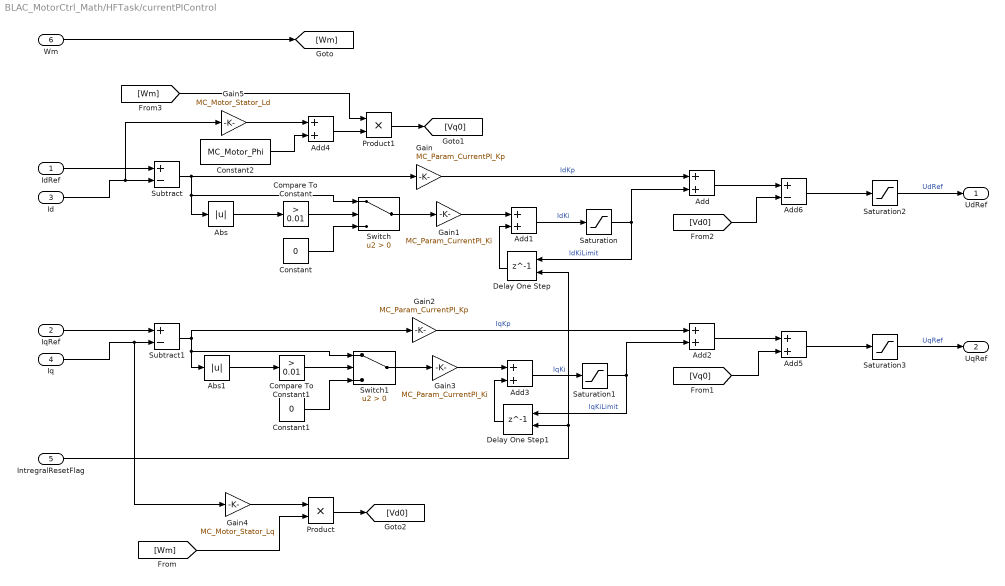
== system BLAC_MotorCtrl_Math/HFTask/currentPIControl ==
  IdRef : Inport
  IqRef : Inport  Port=2
  Id : Inport  Port=3
  Iq : Inport  Port=4
  IntregralResetFlag : Inport  Port=5
  Wm : Inport  Port=6
  Abs : Abs  SaturateOnIntegerOverflow=off
  Abs1 : Abs  SaturateOnIntegerOverflow=off
  Add{,2,4..5} (4 alike) : Sum
  Add1 : Sum  OutDataTypeStr=single
  Add3 : Sum  OutDataTypeStr=single
  Add6 : Sum  Inputs=+-
  Compare To Constant : simulink/Logic and Bit Operations/Compare To Constant  relop=>  const=0.01  OutDataTypeStr=boolean
  Compare To Constant1 : simulink/Logic and Bit Operations/Compare To Constant  relop=>  const=0.01  OutDataTypeStr=boolean
  Constant : Constant  Value=0  OutDataTypeStr=single
  Constant1 : Constant  Value=0  OutDataTypeStr=single
  Constant2 : Constant  Value=MC_Motor_Phi  OutDataTypeStr=single
  Delay One Step : Delay  DelayLength=1  ExternalReset=Level
      settings: InputPortMap=u0,r5
  Delay One Step1 : Delay  DelayLength=1  ExternalReset=Level
      settings: InputPortMap=u0,r5
  Gain : Gain  Gain=MC_Param_CurrentPI_Kp  OutDataTypeStr=single
  Gain1 : Gain  Gain=MC_Param_CurrentPI_Ki  OutDataTypeStr=single
  Gain2 : Gain  Gain=MC_Param_CurrentPI_Kp  OutDataTypeStr=single
  Gain3 : Gain  Gain=MC_Param_CurrentPI_Ki  OutDataTypeStr=single
  Gain4 : Gain  Gain=MC_Motor_Stator_Lq
  Gain5 : Gain  Gain=MC_Motor_Stator_Ld
  Product : Product
  Product1 : Product
  Saturation : Saturate  UpperLimit=MC_Param_CurrentPI_UdInteMax  LowerLimit=MC_Param_CurrentPI_UdInteMin
  Saturation1 : Saturate  UpperLimit=MC_Param_CurrentPI_UqInteMax  LowerLimit=MC_Param_CurrentPI_UqInteMin
  Saturation2 : Saturate  UpperLimit=MC_Param_CurrentPI_UdMax  LowerLimit=MC_Param_CurrentPI_UdMin
  Saturation3 : Saturate  UpperLimit=MC_Param_CurrentPI_UqMax  LowerLimit=MC_Param_CurrentPI_UqMin
  Subtract : Sum  Inputs=+-
  Subtract1 : Sum  Inputs=+-
  Switch : Switch  Criteria=u2 > Threshold  SaturateOnIntegerOverflow=off  InputSameDT=off
  Switch1 : Switch  Criteria=u2 > Threshold  SaturateOnIntegerOverflow=off  InputSameDT=off
  UdRef : Outport
  UqRef : Outport  Port=2
  wires:
  IdRef/1 -> Subtract/1
  Subtract/1 -> Gain/1, Switch/1, Abs/1
  Gain/1 -> Add/1  "IdKp"
  Abs/1 -> Compare To Constant/1
  Gain1/1 -> Add1/1
  Delay One Step/1 -> Add1/2
  Add1/1 -> Saturation/1  "IdKi"
  Saturation/1 -> Add/2, Delay One Step/1  "IdKiLimit"
  Saturation1/1 -> Delay One Step1/1, Add2/2  "IqKiLimit"
  Add3/1 -> Saturation1/1  "IqKi"
  Delay One Step1/1 -> Add3/2
  Gain3/1 -> Add3/1
  Gain2/1 -> Add2/1  "IqKp"
  Subtract1/1 -> Switch1/1, Abs1/1, Gain2/1
  Iq/1 -> Gain4/1, Subtract1/2
  IqRef/1 -> Subtract1/1
  IntregralResetFlag/1 -> Delay One Step/2, Delay One Step1/2
  Add5/1 -> Saturation3/1
  Switch/1 -> Gain1/1
  Compare To Constant/1 -> Switch/2
  Constant/1 -> Switch/3
  Constant1/1 -> Switch1/3
  Compare To Constant1/1 -> Switch1/2
  Abs1/1 -> Compare To Constant1/1
  Switch1/1 -> Gain3/1
  Gain4/1 -> Product/1
  Id/1 -> Gain5/1, Subtract/2
  [Wm] -> Product/2
  Gain5/1 -> Add4/1
  Add4/1 -> Product1/2
  Constant2/1 -> Add4/2
  Product1/1 -> [Vq0]
  Product/1 -> [Vd0]
  Add2/1 -> Add5/1
  [Vq0] -> Add5/2
  Add/1 -> Add6/1
  Add6/1 -> Saturation2/1
  [Vd0] -> Add6/2
  Saturation2/1 -> UdRef/1  "UdRef"
  Saturation3/1 -> UqRef/1  "UqRef"
  [Wm] -> Product1/1
  Wm/1 -> [Wm]

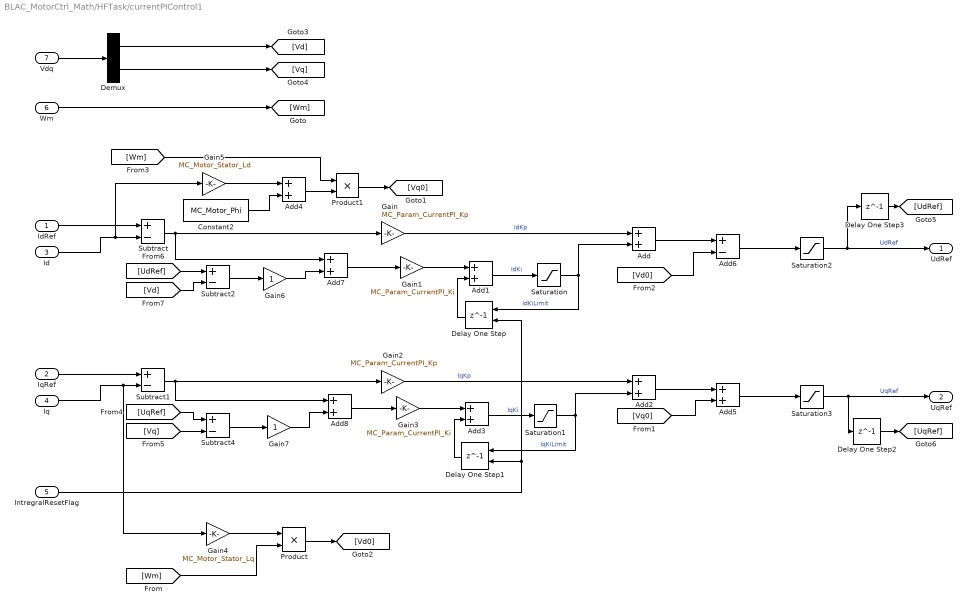
== system BLAC_MotorCtrl_Math/HFTask/currentPIControl1 ==
  IdRef : Inport
  IqRef : Inport  Port=2
  Id : Inport  Port=3
  Iq : Inport  Port=4
  IntregralResetFlag : Inport  Port=5
  Wm : Inport  Port=6
  Vdq : Inport  Port=7
  Add{,2,4..5,7..8} (6 alike) : Sum
  Add1 : Sum  OutDataTypeStr=single
  Add3 : Sum  OutDataTypeStr=single
  Add6 : Sum  Inputs=+-
  Constant2 : Constant  Value=MC_Motor_Phi  OutDataTypeStr=single
  Delay One Step : Delay  DelayLength=1  ExternalReset=Level
      settings: InputPortMap=u0,r5
  Delay One Step1 : Delay  DelayLength=1  ExternalReset=Level
      settings: InputPortMap=u0,r5
  Delay One Step2 : Delay  DelayLength=1  InitialCondition=single(0)
  Delay One Step3 : Delay  DelayLength=1  InitialCondition=single(0)
  Demux : Demux  Outputs=2
  Gain : Gain  Gain=MC_Param_CurrentPI_Kp  OutDataTypeStr=single
  Gain1 : Gain  Gain=MC_Param_CurrentPI_Ki  OutDataTypeStr=single
  Gain2 : Gain  Gain=MC_Param_CurrentPI_Kp  OutDataTypeStr=single
  Gain3 : Gain  Gain=MC_Param_CurrentPI_Ki  OutDataTypeStr=single
  Gain4 : Gain  Gain=MC_Motor_Stator_Lq
  Gain5 : Gain  Gain=MC_Motor_Stator_Ld
  Gain6 : Gain
  Gain7 : Gain
  Product : Product
  Product1 : Product
  Saturation : Saturate  UpperLimit=MC_Param_CurrentPI_UdInteMax  LowerLimit=MC_Param_CurrentPI_UdInteMin
  Saturation1 : Saturate  UpperLimit=MC_Param_CurrentPI_UqInteMax  LowerLimit=MC_Param_CurrentPI_UqInteMin
  Saturation2 : Saturate  UpperLimit=MC_Param_CurrentPI_UdMax  LowerLimit=MC_Param_CurrentPI_UdMin
  Saturation3 : Saturate  UpperLimit=MC_Param_CurrentPI_UqMax  LowerLimit=MC_Param_CurrentPI_UqMin
  Subtract{,1..2,4} (4 alike) : Sum  Inputs=+-
  UdRef : Outport
  UqRef : Outport  Port=2
  wires:
  Wm/1 -> [Wm]
  [Wm] -> Product1/1
  Saturation3/1 -> Delay One Step2/1, UqRef/1  "UqRef"
  Saturation2/1 -> Delay One Step3/1, UdRef/1  "UdRef"
  [Vd0] -> Add6/2
  Add6/1 -> Saturation2/1
  Add/1 -> Add6/1
  [Vq0] -> Add5/2
  Add2/1 -> Add5/1
  Product/1 -> [Vd0]
  Product1/1 -> [Vq0]
  Constant2/1 -> Add4/2
  Add4/1 -> Product1/2
  Gain5/1 -> Add4/1
  [Wm] -> Product/2
  Id/1 -> Subtract/2, Gain5/1
  Gain4/1 -> Product/1
  Add8/1 -> Gain3/1
  Add5/1 -> Saturation3/1
  IntregralResetFlag/1 -> Delay One Step1/2, Delay One Step/2
  IqRef/1 -> Subtract1/1
  Iq/1 -> Subtract1/2, Gain4/1
  Subtract1/1 -> Add8/1, Gain2/1
  Gain2/1 -> Add2/1  "IqKp"
  Gain3/1 -> Add3/1
  Delay One Step1/1 -> Add3/2
  Add3/1 -> Saturation1/1  "IqKi"
  Saturation1/1 -> Add2/2, Delay One Step1/1  "IqKiLimit"
  Saturation/1 -> Delay One Step/1, Add/2  "IdKiLimit"
  Add1/1 -> Saturation/1  "IdKi"
  Delay One Step/1 -> Add1/2
  Gain1/1 -> Add1/1
  Gain/1 -> Add/1  "IdKp"
  Subtract/1 -> Add7/1, Gain/1
  IdRef/1 -> Subtract/1
  Vdq/1 -> Demux/1
  Demux/1 -> [Vd]
  Demux/2 -> [Vq]
  Add7/1 -> Gain1/1
  [Vq] -> Subtract4/2
  [UqRef] -> Subtract4/1
  Subtract2/1 -> Gain6/1
  Gain6/1 -> Add7/2
  Subtract4/1 -> Gain7/1
  Gain7/1 -> Add8/2
  [UdRef] -> Subtract2/1
  [Vd] -> Subtract2/2
  Delay One Step2/1 -> [UqRef]
  Delay One Step3/1 -> [UdRef]

== system BLAC_MotorCtrl_Math/HFTask/currentPIControl2 ==
  IdRef : Inport
  IqRef : Inport  Port=2
  Id : Inport  Port=3
  Iq : Inport  Port=4
  IntregralResetFlag : Inport  Port=5
  Wm : Inport  Port=6
  Abs : Abs  SaturateOnIntegerOverflow=off
  Abs1 : Abs  SaturateOnIntegerOverflow=off
  Add : Sum
  Add1 : Sum  OutDataTypeStr=single
  Add2 : Sum
  Add3 : Sum  OutDataTypeStr=single
  Add4 : Sum  Commented=on
  Add5 : Sum
  Add6 : Sum  Inputs=+-
  Compare To Constant : simulink/Logic and Bit Operations/Compare To Constant  relop=>  const=0.01  OutDataTypeStr=boolean
  Compare To Constant1 : simulink/Logic and Bit Operations/Compare To Constant  relop=>  const=0.01  OutDataTypeStr=boolean
  Constant : Constant  Value=0  OutDataTypeStr=single
  Constant1 : Constant  Value=0  OutDataTypeStr=single
  Constant2 : Constant  Commented=on  Value=MC_Motor_Phi  OutDataTypeStr=single
  Delay One Step : Delay  DelayLength=1  ExternalReset=Level
      settings: InputPortMap=u0,r5
  Delay One Step1 : Delay  DelayLength=1  ExternalReset=Level
      settings: InputPortMap=u0,r5
  From : From  Commented=on  GotoTag=Wm
  From1 : From  Commented=on  GotoTag=Vq0
  From2 : From  Commented=on  GotoTag=Vd0
  From3 : From  Commented=on  GotoTag=Wm
  Gain : Gain  OutDataTypeStr=single
  Gain1 : Gain  Gain=0.01*MC_Sim_HFTStep  OutDataTypeStr=single
  Gain2 : Gain  OutDataTypeStr=single
  Gain3 : Gain  Gain=0.01*MC_Sim_HFTStep  OutDataTypeStr=single
  Gain4 : Gain  Commented=on  Gain=MC_Motor_Stator_Lq
  Gain5 : Gain  Commented=on  Gain=MC_Motor_Stator_Ld
  Goto1 : Goto  Commented=on  GotoTag=Vq0
  Goto2 : Goto  Commented=on  GotoTag=Vd0
  Product : Product  Commented=on
  Product1 : Product  Commented=on
  Saturation : Saturate  UpperLimit=50  LowerLimit=0
  Saturation1 : Saturate  UpperLimit=50  LowerLimit=0
  Saturation2 : Saturate  UpperLimit=300  LowerLimit=0
  Saturation3 : Saturate  UpperLimit=300  LowerLimit=0
  Subtract : Sum  Inputs=+-
  Subtract1 : Sum  Inputs=+-
  Switch : Switch  Criteria=u2 > Threshold  SaturateOnIntegerOverflow=off  InputSameDT=off
  Switch1 : Switch  Criteria=u2 > Threshold  SaturateOnIntegerOverflow=off  InputSameDT=off
  UdRef : Outport
  UqRef : Outport  Port=2
  wires:
  Wm/1 -> [Wm]
  From3/1 -> Product1/1
  Saturation3/1 -> UqRef/1  "UqRef"
  Saturation2/1 -> UdRef/1  "UdRef"
  From2/1 -> Add6/2
  Add6/1 -> Saturation2/1
  Add/1 -> Add6/1
  From1/1 -> Add5/2
  Add2/1 -> Add5/1
  Product/1 -> Goto2/1
  Product1/1 -> Goto1/1
  Constant2/1 -> Add4/2
  Add4/1 -> Product1/2
  Gain5/1 -> Add4/1
  From/1 -> Product/2
  Id/1 -> Subtract/2, Gain5/1
  Gain4/1 -> Product/1
  Switch1/1 -> Gain3/1
  Abs1/1 -> Compare To Constant1/1
  Compare To Constant1/1 -> Switch1/2
  Constant1/1 -> Switch1/3
  Constant/1 -> Switch/3
  Compare To Constant/1 -> Switch/2
  Switch/1 -> Gain1/1
  Add5/1 -> Saturation3/1
  IntregralResetFlag/1 -> Delay One Step1/2, Delay One Step/2
  IqRef/1 -> Subtract1/1
  Iq/1 -> Subtract1/2, Gain4/1
  Subtract1/1 -> Gain2/1, Abs1/1, Switch1/1
  Gain2/1 -> Add2/1  "IqKp"
  Gain3/1 -> Add3/1
  Delay One Step1/1 -> Add3/2
  Add3/1 -> Saturation1/1  "IqKi"
  Saturation1/1 -> Add2/2, Delay One Step1/1  "IqKiLimit"
  Saturation/1 -> Delay One Step/1, Add/2  "IdKiLimit"
  Add1/1 -> Saturation/1  "IdKi"
  Delay One Step/1 -> Add1/2
  Gain1/1 -> Add1/1
  Abs/1 -> Compare To Constant/1
  Gain/1 -> Add/1  "IdKp"
  Subtract/1 -> Abs/1, Switch/1, Gain/1
  IdRef/1 -> Subtract/1

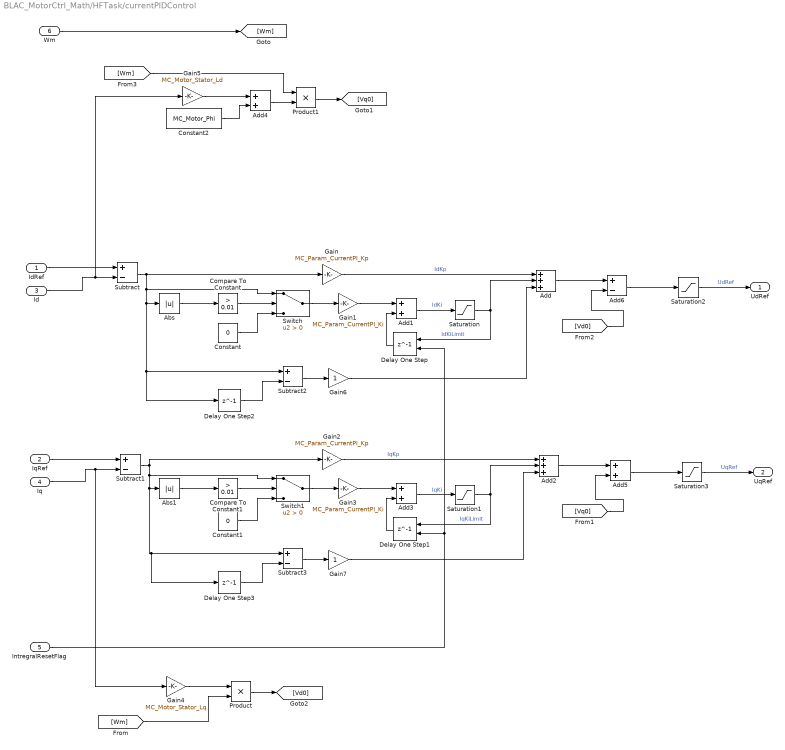
== system BLAC_MotorCtrl_Math/HFTask/currentPIDControl ==
  IdRef : Inport
  IqRef : Inport  Port=2
  Id : Inport  Port=3
  Iq : Inport  Port=4
  IntregralResetFlag : Inport  Port=5
  Wm : Inport  Port=6
  Abs : Abs  SaturateOnIntegerOverflow=off
  Abs1 : Abs  SaturateOnIntegerOverflow=off
  Add : Sum  Inputs=+++
  Add1 : Sum  OutDataTypeStr=single
  Add2 : Sum  Inputs=+++
  Add3 : Sum  OutDataTypeStr=single
  Add4 : Sum
  Add5 : Sum
  Add6 : Sum  Inputs=+-
  Compare To Constant : simulink/Logic and Bit Operations/Compare To Constant  relop=>  const=0.01  OutDataTypeStr=boolean
  Compare To Constant1 : simulink/Logic and Bit Operations/Compare To Constant  relop=>  const=0.01  OutDataTypeStr=boolean
  Constant : Constant  Value=0  OutDataTypeStr=single
  Constant1 : Constant  Value=0  OutDataTypeStr=single
  Constant2 : Constant  Value=MC_Motor_Phi  OutDataTypeStr=single
  Delay One Step : Delay  DelayLength=1  ExternalReset=Level
      settings: InputPortMap=u0,r5
  Delay One Step1 : Delay  DelayLength=1  ExternalReset=Level
      settings: InputPortMap=u0,r5
  Delay One Step2 : Delay  DelayLength=1  InitialCondition=single(0)
  Delay One Step3 : Delay  DelayLength=1  InitialCondition=single(0)
  Gain : Gain  Gain=MC_Param_CurrentPI_Kp  OutDataTypeStr=single
  Gain1 : Gain  Gain=MC_Param_CurrentPI_Ki  OutDataTypeStr=single
  Gain2 : Gain  Gain=MC_Param_CurrentPI_Kp  OutDataTypeStr=single
  Gain3 : Gain  Gain=MC_Param_CurrentPI_Ki  OutDataTypeStr=single
  Gain4 : Gain  Gain=MC_Motor_Stator_Lq
  Gain5 : Gain  Gain=MC_Motor_Stator_Ld
  Gain6 : Gain
  Gain7 : Gain
  Product : Product
  Product1 : Product
  Saturation : Saturate  UpperLimit=MC_Param_CurrentPI_UdInteMax  LowerLimit=MC_Param_CurrentPI_UdInteMin
  Saturation1 : Saturate  UpperLimit=MC_Param_CurrentPI_UqInteMax  LowerLimit=MC_Param_CurrentPI_UqInteMin
  Saturation2 : Saturate  UpperLimit=MC_Param_CurrentPI_UdMax  LowerLimit=MC_Param_CurrentPI_UdMin
  Saturation3 : Saturate  UpperLimit=MC_Param_CurrentPI_UqMax  LowerLimit=MC_Param_CurrentPI_UqMin
  Subtract{,1..3} (4 alike) : Sum  Inputs=+-
  Switch : Switch  Criteria=u2 > Threshold  SaturateOnIntegerOverflow=off  InputSameDT=off
  Switch1 : Switch  Criteria=u2 > Threshold  SaturateOnIntegerOverflow=off  InputSameDT=off
  UdRef : Outport
  UqRef : Outport  Port=2
  wires:
  IdRef/1 -> Subtract/1
  Subtract/1 -> Gain/1, Switch/1, Subtract2/1, Delay One Step2/1, Abs/1
  Gain/1 -> Add/1  "IdKp"
  Abs/1 -> Compare To Constant/1
  Gain1/1 -> Add1/1
  Delay One Step/1 -> Add1/2
  Add1/1 -> Saturation/1  "IdKi"
  Saturation/1 -> Add/2, Delay One Step/1  "IdKiLimit"
  Saturation1/1 -> Delay One Step1/1, Add2/2  "IqKiLimit"
  Add3/1 -> Saturation1/1  "IqKi"
  Delay One Step1/1 -> Add3/2
  Gain3/1 -> Add3/1
  Gain2/1 -> Add2/1  "IqKp"
  Iq/1 -> Subtract1/2, Gain4/1
  IqRef/1 -> Subtract1/1
  IntregralResetFlag/1 -> Delay One Step/2, Delay One Step1/2
  Add5/1 -> Saturation3/1
  Switch/1 -> Gain1/1
  Compare To Constant/1 -> Switch/2
  Constant/1 -> Switch/3
  Constant1/1 -> Switch1/3
  Compare To Constant1/1 -> Switch1/2
  Abs1/1 -> Compare To Constant1/1
  Switch1/1 -> Gain3/1
  Gain4/1 -> Product/1
  Id/1 -> Gain5/1, Subtract/2
  [Wm] -> Product/2
  Gain5/1 -> Add4/1
  Add4/1 -> Product1/2
  Constant2/1 -> Add4/2
  Product1/1 -> [Vq0]
  Product/1 -> [Vd0]
  Add2/1 -> Add5/1
  [Vq0] -> Add5/2
  Add/1 -> Add6/1
  Add6/1 -> Saturation2/1
  [Vd0] -> Add6/2
  Saturation2/1 -> UdRef/1  "UdRef"
  Saturation3/1 -> UqRef/1  "UqRef"
  [Wm] -> Product1/1
  Wm/1 -> [Wm]
  Delay One Step2/1 -> Subtract2/2
  Subtract2/1 -> Gain6/1
  Gain6/1 -> Add/3
  Gain7/1 -> Add2/3
  Subtract3/1 -> Gain7/1
  Delay One Step3/1 -> Subtract3/2
  Subtract1/1 -> Switch1/1, Delay One Step3/1, Subtract3/1, Abs1/1, Gain2/1
